simulink model "simulink_kalmanfilter"  (R2020b)
settings: Solver=ode1  StartTime=0.0  StopTime=inf  FixedStep=0.002  RelTol=1e-3  EnableMultiTasking=on
PostLoadFcn:
  | qc_set_target_type(getConfigSet(bdroot, 'QUARC Default Target Configuration'));
values from neighbouring files (symbols this model uses):
  Ad = sys_disc.A    [init_heli_3_10.m]
  Bd = sys_disc.B    [init_heli_3_10.m]
  Cd = sys_disc.C    [init_heli_3_10.m]
  F = inv((C * inv(B*K - A) * B))    [init_heli_3_10.m]
  Joystick_gain_x = 1    [init_heli_3_10.m]
  Joystick_gain_y = -1    [init_heli_3_10.m]
  K_LQR = lqr(A_aug, B_aug, Q_lqr_aug, R_lqr_aug)    [init_heli_3_10.m]
  k_pd = - (lambda_1 + lambda_2) / K_1    (= 15.5412844037)    [init_heli_3_10.m]
  k_pp = lambda_1 * lambda_2 / K_1    (= 11.3027522936)    [init_heli_3_10.m]
  Qd = [0.0229090668748295,0,0,0,0,0 ... (first row only)    [init_heli_3_10.m]
  Rd = cov_flying    [init_heli_3_10.m]    (also in lab4_cov_calc.m)
  Vs_0 = 7    [init_heli_3_10.m]
undefined symbols (not defined in the file or in its folder): HIL, qc_get_step_size
libraries: quarc_library x9
settings Model: SimulationMode=external  ExtModeTrigDuration=500000  Creator=Rchan  LastModifiedBy=mathskas
settings SolverCC: PositivePriorityOrder=on
settings DataIOCC: LimitDataPoints=on  SaveFormat=Array  SignalLoggingSaveFormat=ModelDataLogs  ReturnWorkspaceOutputs=off
settings OptimizationCC: ExpressionDepthLimit=2147483647  InitFltsAndDblsToZero=on  LifeSpan=inf
settings DebuggingCC: SaveWithParameterizedLinksMsg=none  UnderspecifiedInitializationDetection=Classic  MergeDetectMultiDrivingBlocksExec=none  SolverPrmCheckMsg=warning  MultiTaskDSMMsg=warning  MultiTaskCondExecSysMsg=none  FcnCallInpInsideContextMsg=warning  AllowSymbolicDim=off  StateNameClashWarn=warning  SFUnexpectedBacktrackingDiag=warning  SFNoUnconditionalDefaultTransitionDiag=warning  SFExecutionAtInitializationDiag=none  ArithmeticOperatorsInVariantConditions=warning
settings HardwareCC: ProdBitPerPointer=32  ProdBitPerSizeT=32  ProdBitPerPtrDiffT=32  ProdLargestAtomicFloat=None  ProdIntDivRoundTo=Undefined  ProdEndianess=Unspecified  ProdWordSize=32  ProdHWDeviceType=32-bit Generic
settings ModelReferenceCC: PropagateSignalLabelsOutOfModel=off
settings SFSimCC: SimUseLocalCustomCode=off  CustomCodeUndefinedFunction=UseInterfaceOnly
settings RTWCC: Description=QUARC Win64 Target  SystemTargetFile=quarc_win64.tlc  TemplateMakefile=quarc_default_tmf  RTWUseLocalCustomCode=off
settings CodeAppCC: StateflowObjectComments=on
settings GRTTargetCC: TargetLangStandard=C89/C90 (ANSI)  ParMdlRefBuildCompliant=off  CompOptLevelCompliant=off  CombineOutputUpdateFcns=off  MatFileLogging=off  GRTInterface=on  UseToolchainInfoCompliant=off  ExtMode=on  ExtModeMexFile=quarc_comm
settings ConfigComp: CovMetricSettings=dw  CovSaveCumulativeToWorkspaceVar=on  CovSaveSingleToWorkspaceVar=on  CovExternalEMLEnable=off  CovSFcnEnable=off

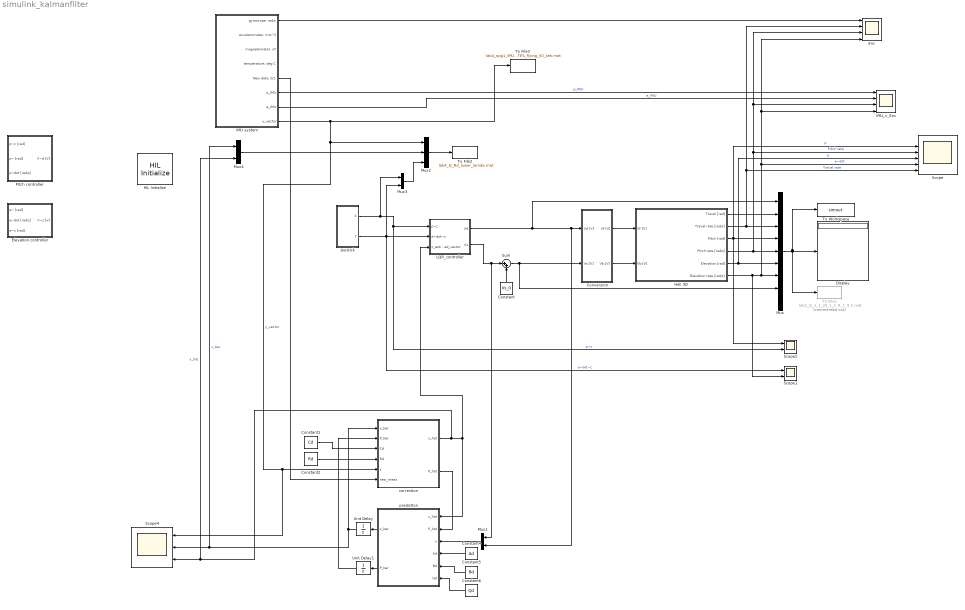
== system simulink_kalmanfilter ==
  Constant : Constant  Value=Vs_0
  Constant1 : Constant  Value=Cd
  Constant2 : Constant  Value=Rd
  Constant4 : Constant  Value=Ad
  Constant5 : Constant  Value=Bd
  Constant6 : Constant  Value=Qd
  Conversion : Subsystem
  Display : Display
  Elevation controller : Subsystem
  Enc : Scope  NumInputPorts=4
  HIL Initialize : quarc_library/Data Acquisition/Generic/Configuration/HIL Initialize  Priority=-99  object_name=HIL-1  board_type=q8_usb  board_number=0  board_options=update_rate=normal;decimation=1  exclusive=off  active=off  hardware_clocks=[0:2]  clock_modes=[]  initial_clock_frequencies=[]  set_clock_params_at_start=off  set_clock_params_at_switch_in=off  set_clock_frequencies_at_start=off  set_clock_frequencies_at_switch_in=off  analog_input_channels=[0:7]  analog_input_configurations=[]  analog_input_maximums=10  analog_input_minimums=-10  set_analog_input_params_at_start=on  set_analog_input_params_at_switch_in=off  analog_output_channels=[0:7]  analog_output_maximums=10  analog_output_minimums=-10  initial_analog_outputs=[0]  final_analog_outputs=[0]  watchdog_analog_outputs=0  set_analog_output_params_at_start=on  set_analog_output_params_at_switch_in=off  set_analog_outputs_at_start=on  set_analog_outputs_at_switch_in=off  set_analog_outputs_at_terminate=on  set_analog_outputs_at_switch_out=off  set_analog_outputs_on_watchdog=off  digital_input_channels=[]  digital_output_channels=[]  digital_output_configuration=[]  initial_digital_outputs=[1]  final_digital_outputs=[1]  watchdog_digital_outputs=[1]  set_digital_output_params_at_start=off  set_digital_output_params_at_switch_in=off  set_digital_outputs_at_start=on  set_digital_outputs_at_switch_in=off  set_digital_outputs_at_terminate=on  set_digital_outputs_at_switch_out=off  set_digital_outputs_on_watchdog=off  encoder_channels=[0:7]  quadrature=[4]  encoder_filter_frequency=[]  initial_encoder_counts=[0]  set_encoder_params_at_start=on  set_encoder_params_at_switch_in=off  set_encoder_counts_at_start=on  set_encoder_counts_at_switch_in=off  pwm_channels=[0:7]  pwm_modes=0  pwm_frequency=99.532799999999995e6/4095  pwm_configuration=[0]  pwm_alignment=[0]  pwm_polarity=[1]  pwm_leading_deadband=[0]  pwm_trailing_deadband=[0]  initial_pwm_outputs=[0]  final_pwm_outputs=[0]  watchdog_pwm_outputs=[0]  set_pwm_params_at_start=on  set_pwm_params_at_switch_in=off  set_pwm_outputs_at_start=on  set_pwm_outputs_at_switch_in=off  set_pwm_outputs_at_terminate=on  set_pwm_outputs_at_switch_out=off  set_pwm_outputs_on_watchdog=off  other_output_channels=[]  initial_other_outputs=[]  final_other_outputs=[]  watchdog_other_outputs=[]  set_other_outputs_at_start=off  set_other_outputs_at_switch_in=off  set_other_outputs_at_terminate=off  set_other_outputs_at_switch_out=off  set_other_outputs_on_watchdog=off
  Heli 3D : Subsystem
  IMU system : Subsystem
  IMU_v_Enc : Scope  NumInputPorts=4
  Joystick : Subsystem
  LQR_controller : Subsystem
  Mux : Mux  Inputs=9
  Mux1 : Mux  Inputs=2
  Mux2 : Mux  Inputs=3
  Mux3 : Mux  Inputs=2
  Mux4 : Mux  Inputs=2
  Pitch controller : Subsystem
  Scope : Scope  NumInputPorts=6
  Scope1 : Scope  NumInputPorts=2
  Scope2 : Scope  NumInputPorts=2
  Scope4 : Scope  NumInputPorts=3
  Sum : Sum  Inputs=|++
  To File1 : ToFile  Commented=on  Filename=lab2_Q_1_1_20_1_1_R_1_0.5.mat
  To File2 : ToFile  Filename=lab4_Q_Rd_lower_lamda.mat
  To File3 : ToFile  Filename=lab4_opg1_IMU_STATES_flying_50_sek.mat
  To Workspace : ToWorkspace  VariableName=simout  SaveFormat=Timeseries  SampleTime=-1
  Unit Delay : UnitDelay  SampleTime=-1  HasFrameUpgradeWarning=on
  Unit Delay1 : UnitDelay  SampleTime=-1  HasFrameUpgradeWarning=on
  correction : MATLAB Function  TreatAsAtomicUnit=on
  prediction : MATLAB Function  TreatAsAtomicUnit=on
  wires:
  Heli 3D/3(Pitch [rad]) -> Scope2/1, Scope/2, Mux/4  "p"
  Heli 3D/4(Pitch rate [rad/s]) -> Mux/5, Scope/3, Enc/3, IMU_v_Enc/3  "Pitch rate"
  Heli 3D/5(Elevation [rad]) -> Scope/4, Mux/6  "e"
  Heli 3D/6(Elevation rate [rad/s]) -> Scope1/2, Scope/5, Enc/4, IMU_v_Enc/4, Mux/7  "e~dot"
  Mux/1 -> Display/1, To Workspace/1, To File1/1
  Constant/1 -> Sum/2
  Sum/1 -> Mux/8, Conversion/2(Vs [V])
  Heli 3D/2(Travel rate [rad/s]) -> Mux/3, Scope/6, Enc/2  "Travel rate"
  Heli 3D/1(Travel [rad]) -> Mux/2
  Joystick/1(X) -> Mux3/1, Scope2/2, LQR_controller/1(p~c)  "p~c"
  Joystick/2(Y) -> Mux3/2, LQR_controller/2(e~dot~c), Scope1/1  "e~dot~c"
  LQR_controller/1(Vd) -> Mux1/2, Conversion/1(Vd [V]), Mux/1
  LQR_controller/2(Vs) -> Mux1/1, Sum/1
  IMU system/6(p_IMU) -> IMU_v_Enc/1  "p_IMU"
  IMU system/7(e_IMU) -> IMU_v_Enc/2  "e_IMU"
  IMU system/8(y_vector) -> To File3/1, Scope4/1, correction/5(y), Mux2/1  "y_vector"
  IMU system/1("gyroscope, rad/s") -> Enc/1
  Mux3/1 -> Mux2/3
  Mux2/1 -> To File2/1
  Conversion/1(Vf [V]) -> Heli 3D/1(Vf [V])
  Conversion/2(Vb [V]) -> Heli 3D/2(Vb [V])
  correction/1(x_hat) -> Scope4/3, Mux4/2, LQR_controller/3(x_estimated_vector), prediction/1(x_hat)  "x_hat"
  correction/2(P_hat) -> prediction/2(P_hat)
  prediction/1(x_bar) -> Unit Delay/1
  prediction/2(P_bar) -> Unit Delay1/1
  Constant4/1 -> prediction/4(Ad)
  Constant5/1 -> prediction/5(Bd)
  Constant6/1 -> prediction/6(Qd)
  Constant1/1 -> correction/3(Cd)
  Constant2/1 -> correction/4(Rd)
  IMU system/5("New data, 0/1") -> correction/6(new_meas)
  Unit Delay/1 -> correction/1(x_bar), Scope4/2, Mux4/1  "x_bar"
  Unit Delay1/1 -> correction/2(P_bar)
  Mux1/1 -> prediction/3(u)
  Mux4/1 -> Mux2/2

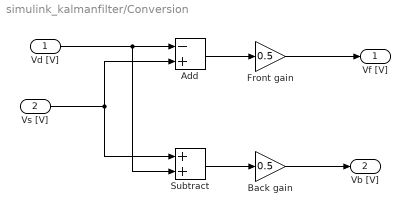
== system simulink_kalmanfilter/Conversion ==
  Vd [V] : Inport
  Vs [V] : Inport  Port=2
  Add : Sum  Inputs=-+
  Back gain : Gain  Gain=0.5
  Front gain : Gain  Gain=0.5
  Subtract : Sum
  Vf [V] : Outport
  Vb [V] : Outport  Port=2
  wires:
  Vd [V]/1 -> Subtract/2, Add/1
  Vs [V]/1 -> Subtract/1, Add/2
  Subtract/1 -> Back gain/1
  Back gain/1 -> Vb [V]/1
  Add/1 -> Front gain/1
  Front gain/1 -> Vf [V]/1

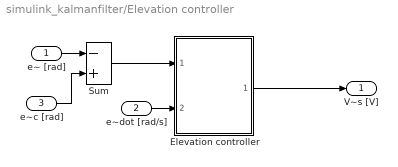
== system simulink_kalmanfilter/Elevation controller ==
  e~ [rad] : Inport
  e~dot [rad/s] : Inport  Port=2
  e~c [rad] : Inport  Port=3
  Elevation controller : Subsystem
  Sum : Sum  Inputs=-+  InputSameDT=on  SaturateOnIntegerOverflow=on  OutDataTypeStr=Inherit: Same as first input
  V~s [V] : Outport  InitialOutput=0
  wires:
  Sum/1 -> Elevation controller/1(e~ [rad])
  Elevation controller/1(V~_s [V]) -> V~s [V]/1
  e~ [rad]/1 -> Sum/1
  e~dot [rad/s]/1 -> Elevation controller/2(e~_dot [rad/s])
  e~c [rad]/1 -> Sum/2

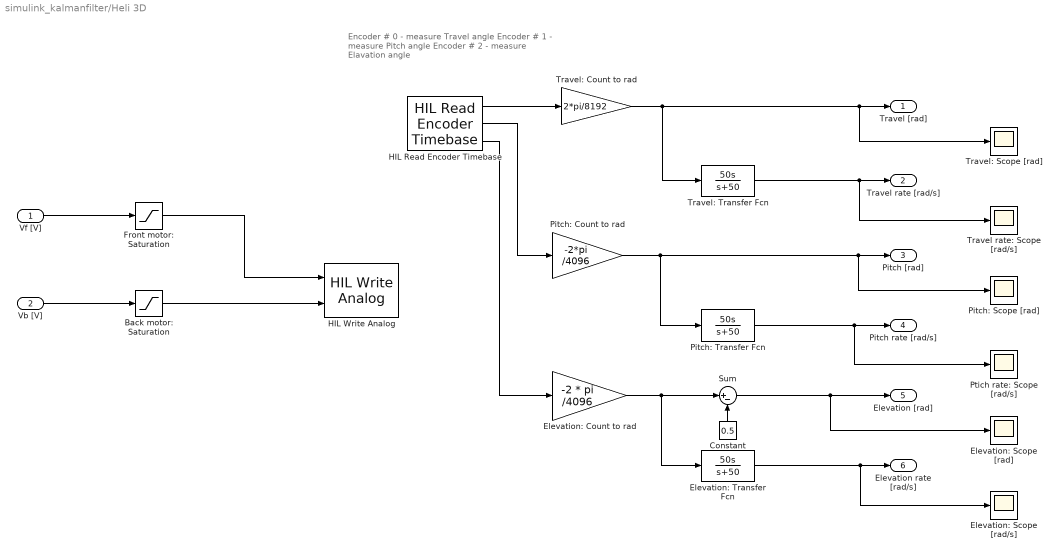
== system simulink_kalmanfilter/Heli 3D ==
  note: Encoder # 0 - measure Travel angle
      | Encoder # 1 - measure Pitch angle
      | Encoder # 2 - measure Elavation angle
  Vf [V] : Inport
  Vb [V] : Inport  Port=2
  Back motor: Saturation : Saturate  UpperLimit=5  LowerLimit=-5
  Constant : Constant  Value=0.5
  Elevation: Count to rad : Gain  Gain=-2 * pi /4096
  Elevation: Scope [rad/s] : Scope
  Elevation: Scope [rad] : Scope
  Elevation: Transfer Fcn : TransferFcn  Numerator=[50 0]  Denominator=[1 50]
  Front motor: Saturation : Saturate  UpperLimit=5  LowerLimit=-5
  HIL Read Encoder Timebase : quarc_library/Data Acquisition/Generic/Timebases/HIL Read Encoder Timebase  object_name=HIL-1  clock=0  channels=[0:2]  active=on  vector_output=off  data_type_mode=Inherit via back propagation  data_type=double  overflow_mode=Error on overflow  samples_in_buffer=max(ceil(1/qc_get_step_size), 1)
  HIL Write Analog : quarc_library/Data Acquisition/Generic/Immediate I//O/HIL Write Analog  object_name=HIL-1  channels=[0:1]  sample_time=-1  active=off  vector_input=off
  Pitch: Count to rad : Gain  Gain=-2*pi /4096
  Pitch: Scope [rad] : Scope
  Pitch: Transfer Fcn : TransferFcn  Numerator=[50 0]  Denominator=[1 50]
  Ptich rate: Scope [rad/s] : Scope
  Sum : Sum  Inputs=|+-
  Travel rate: Scope [rad/s] : Scope
  Travel: Count to rad : Gain  Gain=2*pi/8192
  Travel: Scope [rad] : Scope
  Travel: Transfer Fcn : TransferFcn  Numerator=[50 0]  Denominator=[1 50]
  Travel [rad] : Outport
  Travel rate [rad/s] : Outport  Port=2
  Pitch [rad] : Outport  Port=3
  Pitch rate [rad/s] : Outport  Port=4
  Elevation [rad] : Outport  Port=5
  Elevation rate [rad/s] : Outport  Port=6
  wires:
  HIL Read Encoder Timebase/1 -> Travel: Count to rad/1
  HIL Read Encoder Timebase/2 -> Pitch: Count to rad/1
  HIL Read Encoder Timebase/3 -> Elevation: Count to rad/1
  Travel: Count to rad/1 -> Travel: Scope [rad]/1, Travel [rad]/1, Travel: Transfer Fcn/1
  Travel: Transfer Fcn/1 -> Travel rate: Scope [rad/s]/1, Travel rate [rad/s]/1
  Pitch: Count to rad/1 -> Pitch: Transfer Fcn/1, Pitch: Scope [rad]/1, Pitch [rad]/1
  Pitch: Transfer Fcn/1 -> Ptich rate: Scope [rad/s]/1, Pitch rate [rad/s]/1
  Elevation: Transfer Fcn/1 -> Elevation: Scope [rad/s]/1, Elevation rate [rad/s]/1
  Vf [V]/1 -> Front motor: Saturation/1
  Vb [V]/1 -> Back motor: Saturation/1
  Front motor: Saturation/1 -> HIL Write Analog/1
  Back motor: Saturation/1 -> HIL Write Analog/2
  Elevation: Count to rad/1 -> Elevation: Transfer Fcn/1, Sum/1
  Sum/1 -> Elevation: Scope [rad]/1, Elevation [rad]/1
  Constant/1 -> Sum/2

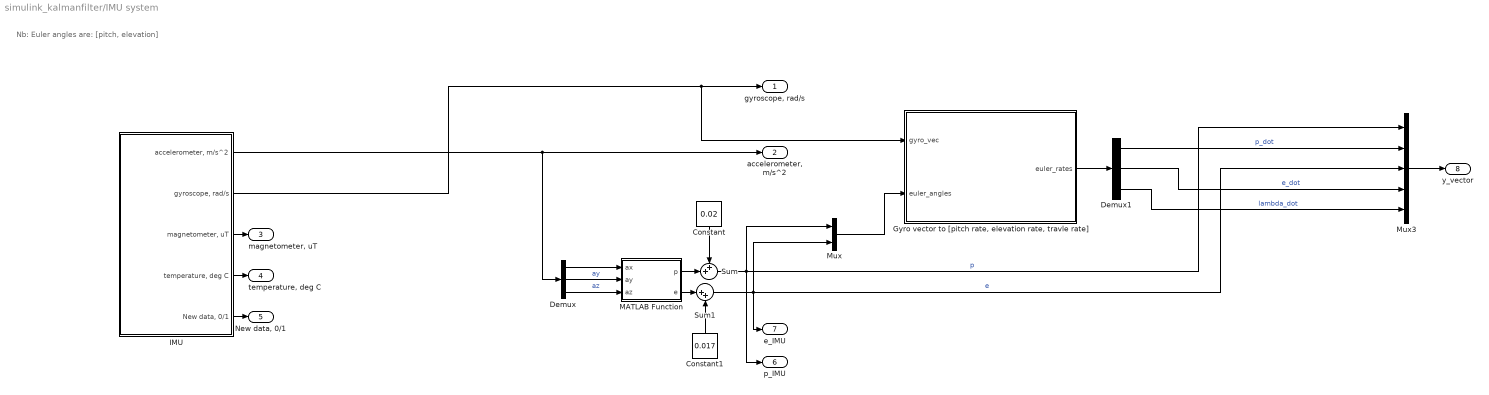
== system simulink_kalmanfilter/IMU system ==
  note: Nb: Euler angles are: [pitch, elevation]
  Constant : Constant  Value=0.02
  Constant1 : Constant  Value=0.017
  Demux : Demux  Outputs=3
  Demux1 : Demux  Outputs=3
  "Gyro vector to [pitch rate, elevation rate, travle rate]" : MATLAB Function  TreatAsAtomicUnit=on
  IMU : Subsystem
  MATLAB Function : MATLAB Function  TreatAsAtomicUnit=on
  Mux : Mux  Inputs=2
  Mux3 : Mux  Inputs=5
  Sum : Sum  Inputs=++|
  Sum1 : Sum  Inputs=|++
  "gyroscope, rad/s" : Outport
  "accelerometer, m/s^2" : Outport  Port=2
  "magnetometer, uT" : Outport  Port=3
  "temperature, deg C" : Outport  Port=4
  "New data, 0/1" : Outport  Port=5
  p_IMU : Outport  Port=6
  e_IMU : Outport  Port=7
  y_vector : Outport  Port=8
  wires:
  IMU/5("New data, 0/1") -> "New data, 0/1"/1
  IMU/3("magnetometer, uT") -> "magnetometer, uT"/1
  IMU/2("gyroscope, rad/s") -> "Gyro vector to [pitch rate, elevation rate, travle rate]"/1(gyro_vec), "gyroscope, rad/s"/1
  IMU/1("accelerometer, m/s^2") -> Demux/1, "accelerometer, m/s^2"/1
  IMU/4("temperature, deg C") -> "temperature, deg C"/1
  Demux/1 -> MATLAB Function/1(ax)
  Demux/2 -> MATLAB Function/2(ay)  "ay"
  Demux/3 -> MATLAB Function/3(az)  "az"
  Mux/1 -> "Gyro vector to [pitch rate, elevation rate, travle rate]"/2(euler_angles)
  MATLAB Function/1(p) -> Sum/2
  Sum/1 -> p_IMU/1, Mux3/1, Mux/1  "p"
  Constant/1 -> Sum/1
  MATLAB Function/2(e) -> Sum1/1
  Sum1/1 -> Mux/2, Mux3/3, e_IMU/1  "e"
  Constant1/1 -> Sum1/2
  "Gyro vector to [pitch rate, elevation rate, travle rate]"/1(euler_rates) -> Demux1/1
  Demux1/2 -> Mux3/4  "e_dot"
  Demux1/1 -> Mux3/2  "p_dot"
  Demux1/3 -> Mux3/5  "lambda_dot"
  Mux3/1 -> y_vector/1

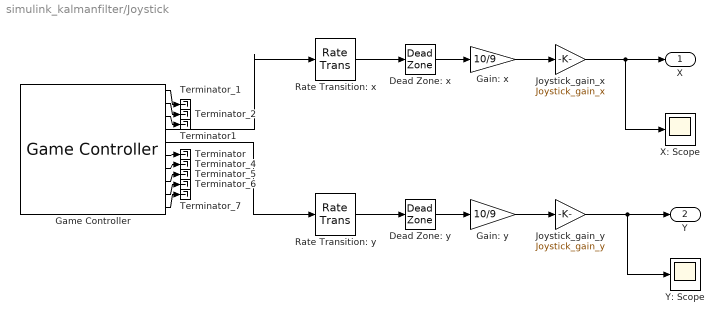
== system simulink_kalmanfilter/Joystick ==
  Dead Zone: x : DeadZone  LowerValue=-0.1  UpperValue=0.1  SaturateOnIntegerOverflow=on
  Dead Zone: y : DeadZone  LowerValue=-0.1  UpperValue=0.1  SaturateOnIntegerOverflow=on
  Gain: x : Gain  Gain=10/9
  Gain: y : Gain  Gain=10/9
  Game Controller : quarc_library/Devices/Peripherals/Target/Game Controller  controller=1  buffer_size=12  deadzone=[]  saturation=[]  sample_time=max(qc_get_step_size, 0.01)  auto_center=off  enabled=on
      settings: SourceProductName=QUARC Targets
  Joystick_gain_x : Gain  Gain=Joystick_gain_x
  Joystick_gain_y : Gain  Gain=Joystick_gain_y
  Rate Transition: x : RateTransition
  Rate Transition: y : RateTransition
  Terminator : Terminator
  Terminator1 : Terminator
  Terminator_{1..2,4..7} (6 alike) : Terminator
  X: Scope : Scope
  Y: Scope : Scope
  X : Outport
  Y : Outport  Port=2
  wires:
  Rate Transition: y/1 -> Dead Zone: y/1
  Rate Transition: x/1 -> Dead Zone: x/1
  Game Controller/5 -> Rate Transition: y/1
  Game Controller/4 -> Rate Transition: x/1
  Game Controller/1 -> Terminator_1/1
  Game Controller/2 -> Terminator_2/1
  Game Controller/7 -> Terminator_4/1
  Game Controller/8 -> Terminator_5/1
  Game Controller/9 -> Terminator_6/1
  Game Controller/10 -> Terminator_7/1
  Game Controller/3 -> Terminator1/1
  Game Controller/6 -> Terminator/1
  Dead Zone: x/1 -> Gain: x/1
  Dead Zone: y/1 -> Gain: y/1
  Gain: x/1 -> Joystick_gain_x/1
  Gain: y/1 -> Joystick_gain_y/1
  Joystick_gain_x/1 -> X/1, X: Scope/1
  Joystick_gain_y/1 -> Y: Scope/1, Y/1

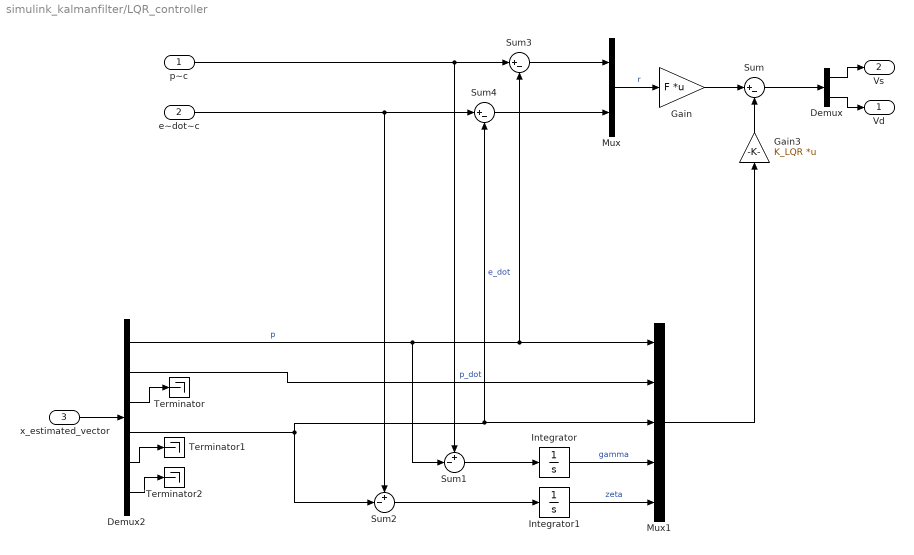
== system simulink_kalmanfilter/LQR_controller ==
  p~c : Inport
  e~dot~c : Inport  Port=2
  x_estimated_vector : Inport  Port=3
  Demux : Demux  Outputs=2
  Demux2 : Demux  Outputs=6
  Gain : Gain  Gain=F  Multiplication=Matrix(K*u)
  Gain3 : Gain  Gain=K_LQR  Multiplication=Matrix(K*u)
  Integrator : Integrator
  Integrator1 : Integrator
  Mux : Mux  Inputs=2
  Mux1 : Mux  Inputs=5
  Sum : Sum  Inputs=|+-
  Sum1 : Sum  Inputs=+-|
  Sum2 : Sum  Inputs=+-|
  Sum3 : Sum  Inputs=|+-
  Sum4 : Sum  Inputs=|+-
  Terminator : Terminator
  Terminator1 : Terminator
  Terminator2 : Terminator
  Vd : Outport
  Vs : Outport  Port=2
  wires:
  e~dot~c/1 -> Sum2/1, Sum4/1
  Mux/1 -> Gain/1  "r"
  Gain3/1 -> Sum/2
  Gain/1 -> Sum/1
  Sum/1 -> Demux/1
  Demux/1 -> Vs/1
  Demux/2 -> Vd/1
  Mux1/1 -> Gain3/1
  Sum1/1 -> Integrator/1
  Integrator/1 -> Mux1/4  "gamma"
  Integrator1/1 -> Mux1/5  "zeta"
  Sum2/1 -> Integrator1/1
  x_estimated_vector/1 -> Demux2/1
  Sum3/1 -> Mux/1
  Sum4/1 -> Mux/2
  Demux2/1 -> Sum1/2, Mux1/1, Sum3/2  "p"
  Demux2/2 -> Mux1/2  "p_dot"
  Demux2/4 -> Mux1/3, Sum4/2, Sum2/2  "e_dot"
  p~c/1 -> Sum1/1, Sum3/1
  Demux2/3 -> Terminator/1
  Demux2/5 -> Terminator1/1
  Demux2/6 -> Terminator2/1

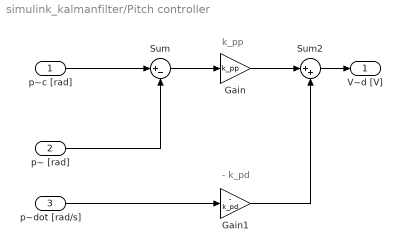
== system simulink_kalmanfilter/Pitch controller ==
  note: k_pp
  note: - k_pd
  p~c [rad] : Inport
  p~ [rad] : Inport  Port=2
  p~dot [rad/s] : Inport  Port=3
  Gain : Gain  Gain=k_pp
  Gain1 : Gain  Gain=- k_pd
  Sum : Sum  Inputs=|+-
  Sum2 : Sum  Inputs=|++
  V~d [V] : Outport  InitialOutput=0
  wires:
  p~c [rad]/1 -> Sum/1
  p~ [rad]/1 -> Sum/2
  Sum2/1 -> V~d [V]/1
  Sum/1 -> Gain/1
  Gain/1 -> Sum2/1
  p~dot [rad/s]/1 -> Gain1/1
  Gain1/1 -> Sum2/2

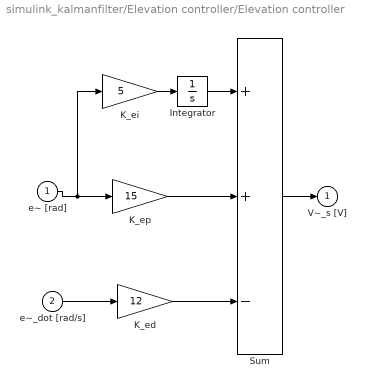
== system simulink_kalmanfilter/Elevation controller/Elevation controller ==
  e~ [rad] : Inport
  e~_dot [rad/s] : Inport  Port=2
  Integrator : Integrator  LimitOutput=on
  K_ed : Gain  Gain=12  SaturateOnIntegerOverflow=on  OutDataTypeStr=Inherit: Same as input  ParamDataTypeStr=Inherit: Same as input
  K_ei : Gain  Gain=5  SaturateOnIntegerOverflow=on  OutDataTypeStr=Inherit: Same as input  ParamDataTypeStr=Inherit: Same as input
  K_ep : Gain  Gain=15  SaturateOnIntegerOverflow=on  OutDataTypeStr=Inherit: Same as input  ParamDataTypeStr=Inherit: Same as input
  Sum : Sum  Inputs=++-  InputSameDT=on  SaturateOnIntegerOverflow=on  OutDataTypeStr=Inherit: Same as first input
  V~_s [V] : Outport  InitialOutput=0
  wires:
  K_ei/1 -> Integrator/1
  Integrator/1 -> Sum/1
  Sum/1 -> V~_s [V]/1
  e~_dot [rad/s]/1 -> K_ed/1
  K_ed/1 -> Sum/3
  K_ep/1 -> Sum/2
  e~ [rad]/1 -> K_ep/1, K_ei/1

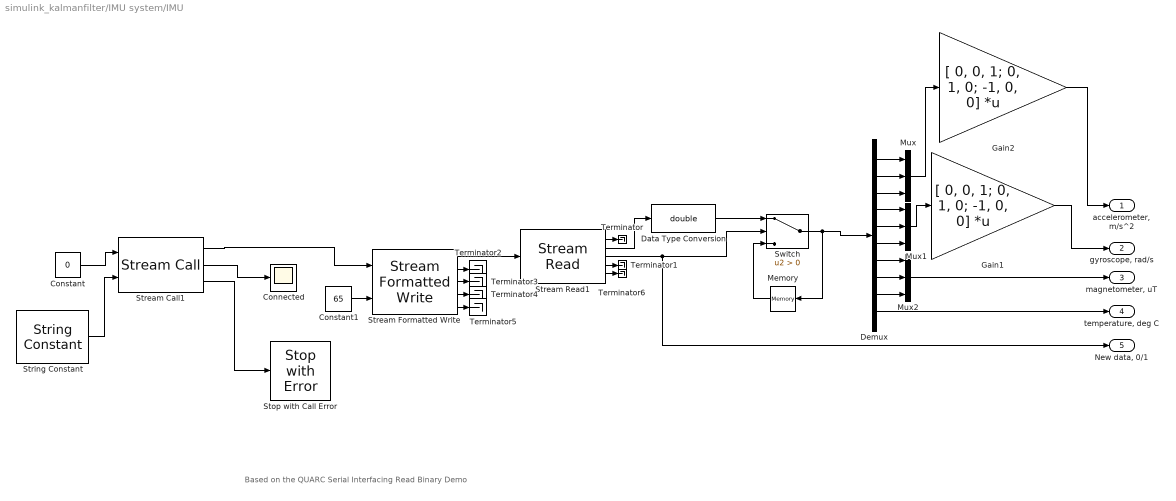
== system simulink_kalmanfilter/IMU system/IMU ==
  note: Based on the QUARC Serial Interfacing Read Binary Demo
  Connected : Scope
  Constant : Constant  Value=0
  Constant1 : Constant  Value=65
  Data Type Conversion : DataTypeConversion  OutDataTypeStr=double
  Demux : Demux  Outputs=10
  Gain1 : Gain  Gain=[ 0, 0, 1; 0, 1, 0; -1, 0, 0]  Multiplication=Matrix(K*u) (u vector)
  Gain2 : Gain  Gain=[ 0, 0, 1; 0, 1, 0; -1, 0, 0]  Multiplication=Matrix(K*u) (u vector)
  Memory : Memory  InitialCondition=[0 0 0 0 0 0 0 0 0 0]
  Mux : Mux  Inputs=3
  Mux1 : Mux  Inputs=3
  Mux2 : Mux  Inputs=3
  Stop with Call Error : quarc_library/Sinks/Error Handling/Stop with Error  message_type=Interpret input as error code  message=Error occurred
      settings: SourceProductName=QUARC Targets
  Stream Call1 : quarc_library/Communications/Intermediate/Stream Call  uri_source=External input port  uri=serial://IMU:9?baud=115200,word=8,parity=none,stop=1,flow='none'  apply_uri_to_all_configs=on  send_buffer_size=8000  receive_buffer_size=8000  byte_order=little endian (Intel - LSB first)  sample_time=qc_get_step_size  non_blocking=on  active=off
      settings: SourceProductName=QUARC Targets
  Stream Formatted Write : quarc_library/Communications/Intermediate/Stream Formatted Write  format_string=%c\n  max_code_units=80  optimization=Minimizing latency
      settings: SourceProductName=QUARC Targets
  Stream Read1 : quarc_library/Communications/Intermediate/Stream Read  data_type=single  type_expr=BusObject  num_elements=10  receive_dims=off
      settings: SourceProductName=QUARC Targets
  String Constant : quarc_library/Strings/String Constant  string_value=qc_perform_substitutions('serial://IMU:%{PORT}?baud=115200,word=8,parity=none,stop=1')  evaluate_string=on  string_type=URI  max_length=255  sample_time=inf  variable_size=off
      settings: AttributesFormatString="\"serial://IMU:3?baud=115200,word=8,parity=none,stop=1\""  SourceProductName=QUARC Targets
  Switch : Switch  Criteria=u2 > Threshold
  Terminator{,1..6} (7 alike) : Terminator
  "accelerometer, m/s^2" : Outport
  "gyroscope, rad/s" : Outport  Port=2
  "magnetometer, uT" : Outport  Port=3
  "temperature, deg C" : Outport  Port=4
  "New data, 0/1" : Outport  Port=5
  wires:
  Switch/1 -> Memory/1, Demux/1
  Data Type Conversion/1 -> Switch/1
  Stream Read1/3 -> "New data, 0/1"/1, Switch/2
  Stream Formatted Write/1 -> Stream Read1/1
  Constant1/1 -> Stream Formatted Write/2
  Gain1/1 -> "gyroscope, rad/s"/1
  Gain2/1 -> "accelerometer, m/s^2"/1
  Stream Read1/4 -> Terminator1/1
  Demux/10 -> "temperature, deg C"/1
  Mux1/1 -> Gain1/1
  Stream Read1/2 -> Data Type Conversion/1
  Demux/7 -> Mux2/1
  Demux/8 -> Mux2/2
  Demux/9 -> Mux2/3
  Mux2/1 -> "magnetometer, uT"/1
  Demux/6 -> Mux1/3
  Demux/5 -> Mux1/2
  Demux/4 -> Mux1/1
  Mux/1 -> Gain2/1
  Demux/3 -> Mux/3
  Demux/1 -> Mux/1
  Demux/2 -> Mux/2
  Stream Read1/1 -> Terminator/1
  Stream Call1/1 -> Stream Formatted Write/1
  Constant/1 -> Stream Call1/1
  String Constant/1 -> Stream Call1/2
  Stream Call1/2 -> Connected/1
  Stream Call1/3 -> Stop with Call Error/1
  Memory/1 -> Switch/3
  Stream Formatted Write/2 -> Terminator2/1
  Stream Formatted Write/3 -> Terminator3/1
  Stream Formatted Write/4 -> Terminator4/1
  Stream Formatted Write/5 -> Terminator5/1
  Stream Read1/5 -> Terminator6/1

== matlab function simulink_kalmanfilter/IMU system/MATLAB Function ==
  data: ax input; p output; e output; ay input; az input
function [p, e] = fcn(ax, ay, az)
if az == 0
    az = 0.01;
    if ay == 0
        ay = 0.01;
    end
end
e = atan(ax/(sqrt(ay^2 + az^2)));
p = atan(ay/az);

== matlab function simulink_kalmanfilter/IMU system/Gyro vector to [pitch rate, elevation rate, travle rate] ==
  data: gyro_vec input; euler_rates output; euler_angles input
function euler_rates = gyro_vec_to_euler_rates(gyro_vec,euler_angles)
%#codegen
    phi = euler_angles(1);
    theta = euler_angles(2);
    %psi = euler_angles(3);


    T = [1, sin(phi)*tan(theta), cos(phi)*tan(theta);
         0, cos(phi),            -sin(phi);
         0, sin(phi)/cos(theta), cos(phi)/cos(theta)]; 
euler_rates = T*gyro_vec;

== matlab function simulink_kalmanfilter/correction ==
  data: x_bar input size=[6,1]; P_bar input size=[6,6]; x_hat output size=[6,1]; Cd input size=[5,6]; Rd input size=[5,5]; y input size=[5,1]; new_meas input; P_hat output size=[6,6]
function [x_hat, P_hat] = correction(x_bar, P_bar, Cd, Rd, y, new_meas)
  if new_meas
      L = P_bar * Cd' * inv(Cd * P_bar * Cd' + Rd);
      x_hat = x_bar + L * (y - Cd*x_bar);
      P_hat = (eye(6) - L*Cd) * P_bar * (eye(6) - L*Cd)' + L * Rd * L';
  else
      x_hat = x_bar;
      P_hat = P_bar;
  end

== matlab function simulink_kalmanfilter/prediction ==
  data: x_hat input size=[6,1]; P_hat input size=[6,6]; u input; x_bar output size=[6,1]; Ad input size=[6,6]; Bd input; Qd input size=[6,6]; P_bar output size=[6,6]
function [x_bar, P_bar] = fcn(x_hat, P_hat, u, Ad, Bd, Qd)
    x_bar = Ad * x_hat + Bd * u;
    P_bar = Ad * P_hat * Ad' + Qd;
end
